simulink model "FM_Transmission_Reception_System"  (R2024a)
settings: Solver=VariableStepAuto  StartTime=0.0  StopTime=10.0  RelTol=1e-3
undefined symbols (not defined in the file): DiscIntNeverNeededParam
libraries: dspstat3 x4, dspfdesign x3, dspmathops x2, dspsrcs4 x1
settings Model: Creator=pyrpo  LastModifiedBy=pyrpo

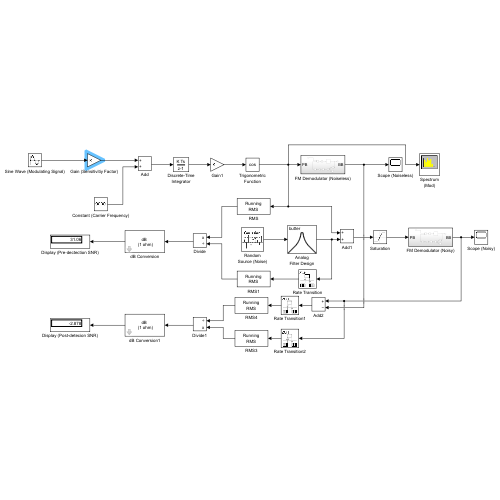
[thumbnail: Simulink's stored preview of the top-level diagram]
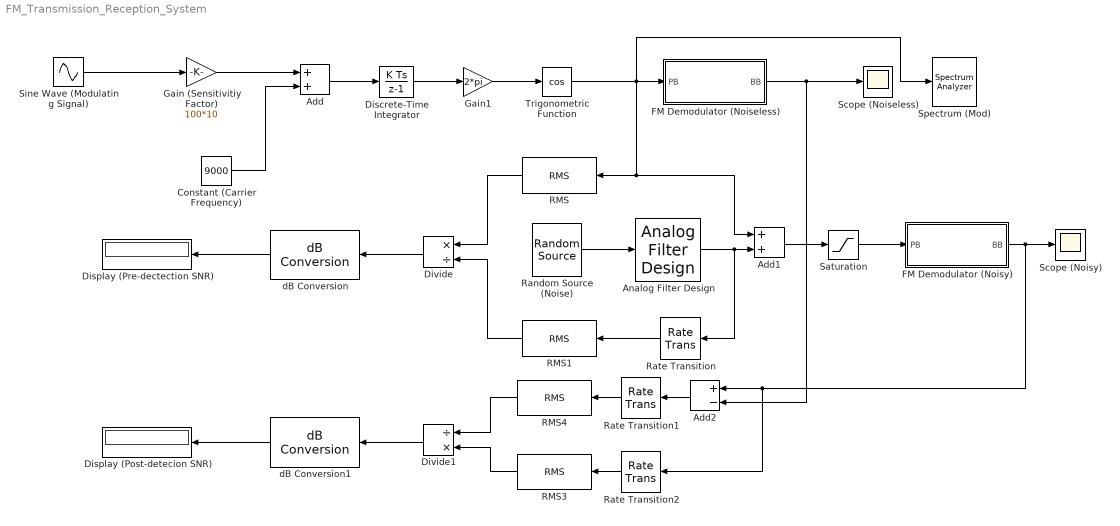
== system FM_Transmission_Reception_System ==
  Add : Sum
  Add1 : Sum
  Add2 : Sum  Inputs=+-
  Analog Filter Design : dspfdesign/Analog Filter Design  method=Butterworth  filttype=Bandpass  N=8  Wlo=8000*2*pi  Whi=10000*2*pi  Rp=2  Rs=40
  Constant (Carrier Frequency) : Constant  Value=9000
  Discrete-Time Integrator : DiscreteIntegrator  SampleTime=1e-5  ICPrevOutput=DiscIntNeverNeededParam  ICPrevScaledInput=DiscIntNeverNeededParam
  Display (Post-detecion SNR) : Display
  Display (Pre-dectection SNR) : Display
  Divide : Product  Inputs=*/
  Divide1 : Product  Inputs=/*
  FM Demodulator (Noiseless) : Subsystem
  FM Demodulator (Noisy) : Subsystem
  Gain (Sensitivitiy Factor) : Gain  Gain=100*10
  Gain1 : Gain  Gain=2*pi
  RMS{,1,3..4} (4 alike) : dspstat3/RMS  run=on  directionMode=Each column  dimension=1  InputProcessing=Columns as channels (frame based)  reset_popup=None
  Random Source (Noise) : dspsrcs4/Random Source  SrcType=Gaussian  MinVal=0  MaxVal=1  MeanVal=0  VarVal=1e-2  RepMode=Specify seed  rawSeed=1  IsInherit=off  SampTime=1e-5  SampFrame=1  OutComplex=Real  DataType=double  SimulateUsing=Interpreted execution
  Rate Transition : RateTransition  OutPortSampleTime=1e-5
  Rate Transition1 : RateTransition  OutPortSampleTime=1e-5
  Rate Transition2 : RateTransition  OutPortSampleTime=1e-5
  Saturation : Saturate  UpperLimit=1  LowerLimit=-1
  Scope (Noiseless) : Scope
  Scope (Noisy) : Scope
  Sine Wave (Modulating Signal) : Sin  SineType=Sample based  Samples=1000  SampleTime=1e-5
  Spectrum (Mod) : SpectrumAnalyzer  WindowPosition=[1.000000,49.000000,1536.000000,792.000000,]  Visible=on  ScopeFrameLocation=window  PlotAsTwoSidedSpectrum=off  RBWSource=Property  RBW=1  Span=49999.99999999999  CenterFrequency=24999.999999999996  StartFrequency=0  StopFrequency=49999.99999999999  YLimits=[-255.4566928823593,82.82456219997775]  ShowLegend=on  SelectedToolstripTab=spectrumAnalyzerToolstrip.channelMeasurementsTab
  Trigonometric Function : Trigonometry  Operator=cos
  dB Conversion : dspmathops/dB Conversion  dBtype=dB  intype=Amplitude  R=1  fuzz=off
      settings: LibrarySourceBlock=commutil2/dB Conversion
  dB Conversion1 : dspmathops/dB Conversion  dBtype=dB  intype=Amplitude  R=1  fuzz=off
      settings: LibrarySourceBlock=commutil2/dB Conversion
  wires:
  Sine Wave (Modulating Signal)/1 -> Gain (Sensitivitiy Factor)/1
  Gain (Sensitivitiy Factor)/1 -> Add/1
  Constant (Carrier Frequency)/1 -> Add/2
  Add/1 -> Discrete-Time Integrator/1
  Discrete-Time Integrator/1 -> Gain1/1
  Gain1/1 -> Trigonometric Function/1
  Trigonometric Function/1 -> Spectrum (Mod)/1, FM Demodulator (Noiseless)/1(PB), RMS/1, Add1/1
  FM Demodulator (Noiseless)/1(BB) -> Scope (Noiseless)/1, Add2/2
  dB Conversion/1 -> Display (Pre-dectection SNR)/1
  Divide/1 -> dB Conversion/1
  RMS/1 -> Divide/1
  RMS1/1 -> Divide/2
  Add2/1 -> Rate Transition1/1
  Rate Transition1/1 -> RMS4/1
  Rate Transition/1 -> RMS1/1
  Random Source (Noise)/1 -> Analog Filter Design/1
  Analog Filter Design/1 -> Rate Transition/1, Add1/2
  Add1/1 -> Saturation/1
  Rate Transition2/1 -> RMS3/1
  RMS3/1 -> Divide1/2
  RMS4/1 -> Divide1/1
  Divide1/1 -> dB Conversion1/1
  dB Conversion1/1 -> Display (Post-detecion SNR)/1
  Saturation/1 -> FM Demodulator (Noisy)/1(PB)
  FM Demodulator (Noisy)/1(BB) -> Add2/1, Rate Transition2/1, Scope (Noisy)/1

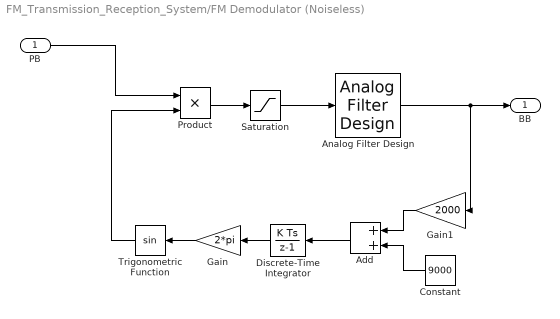
== system FM_Transmission_Reception_System/FM Demodulator (Noiseless) ==
  PB : Inport
  Add : Sum
  Analog Filter Design : dspfdesign/Analog Filter Design  method=Butterworth  filttype=Lowpass  N=8  Wlo=200*2*pi  Whi=80  Rp=2  Rs=40
  Constant : Constant  Value=9000
  Discrete-Time Integrator : DiscreteIntegrator  SampleTime=1e-5  ICPrevOutput=DiscIntNeverNeededParam  ICPrevScaledInput=DiscIntNeverNeededParam
  Gain : Gain  Gain=2*pi
  Gain1 : Gain  Gain=2000
  Product : Product
  Saturation : Saturate
  Trigonometric Function : Trigonometry
  BB : Outport
  wires:
  PB/1 -> Product/1
  Product/1 -> Saturation/1
  Saturation/1 -> Analog Filter Design/1
  Analog Filter Design/1 -> Gain1/1, BB/1
  Constant/1 -> Add/2
  Gain1/1 -> Add/1
  Add/1 -> Discrete-Time Integrator/1
  Discrete-Time Integrator/1 -> Gain/1
  Gain/1 -> Trigonometric Function/1
  Trigonometric Function/1 -> Product/2

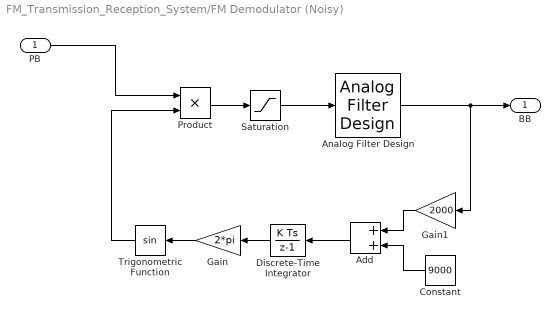
== system FM_Transmission_Reception_System/FM Demodulator (Noisy) ==
  PB : Inport
  Add : Sum
  Analog Filter Design : dspfdesign/Analog Filter Design  method=Butterworth  filttype=Lowpass  N=8  Wlo=200*2*pi  Whi=80  Rp=2  Rs=40
  Constant : Constant  Value=9000
  Discrete-Time Integrator : DiscreteIntegrator  SampleTime=1e-5  ICPrevOutput=DiscIntNeverNeededParam  ICPrevScaledInput=DiscIntNeverNeededParam
  Gain : Gain  Gain=2*pi
  Gain1 : Gain  Gain=2000
  Product : Product
  Saturation : Saturate
  Trigonometric Function : Trigonometry
  BB : Outport
  wires:
  Trigonometric Function/1 -> Product/2
  Saturation/1 -> Analog Filter Design/1
  Constant/1 -> Add/2
  Gain1/1 -> Add/1
  Add/1 -> Discrete-Time Integrator/1
  Gain/1 -> Trigonometric Function/1
  Product/1 -> Saturation/1
  Analog Filter Design/1 -> Gain1/1, BB/1
  PB/1 -> Product/1
  Discrete-Time Integrator/1 -> Gain/1
